simulink model "matrixMultEigenText"  (R2013b)
settings: Solver=ode3  StartTime=0.0  StopTime=10.0  FixedStep=0.001  RelTol=1e-3
InitFcn:
  | dim = 8;
  | a=randn(dim,dim);
  | matrix = ss(-a*a',randn(dim,1),randn(1,dim),0);
  | 
  | dim2 = 1;
  | dim3 = 2;
  | matA = randn(dim,dim2);
  | matC = randn(dim2,dim2);
  | matB = randn(dim2,dim3);
settings Model: Creator=rtai-ao  LastModifiedBy=rtai-ao
settings DebuggingCC: ModelReferenceIOMismatchMessage=warning
settings RTWCC: SystemTargetFile=rtai.tlc  TemplateMakefile=rtai.tmf  Description=Linux RTAI Real-Time Target  GenerateReport=on  ProcessScript=rtai_make_rtw_hook  BuildConfiguration=Faster Runs
settings STFCustomTargetCC: ModelReferenceCompliant=off  GeneratePreprocessorConditionals=Disable all  MatFileLogging=on  MATLABClassNameForMDSCustomization=Simulink.SoftwareTarget.TargetSpecificTriggerConfigurationBase  SystemTargetFile=rtai.tlc

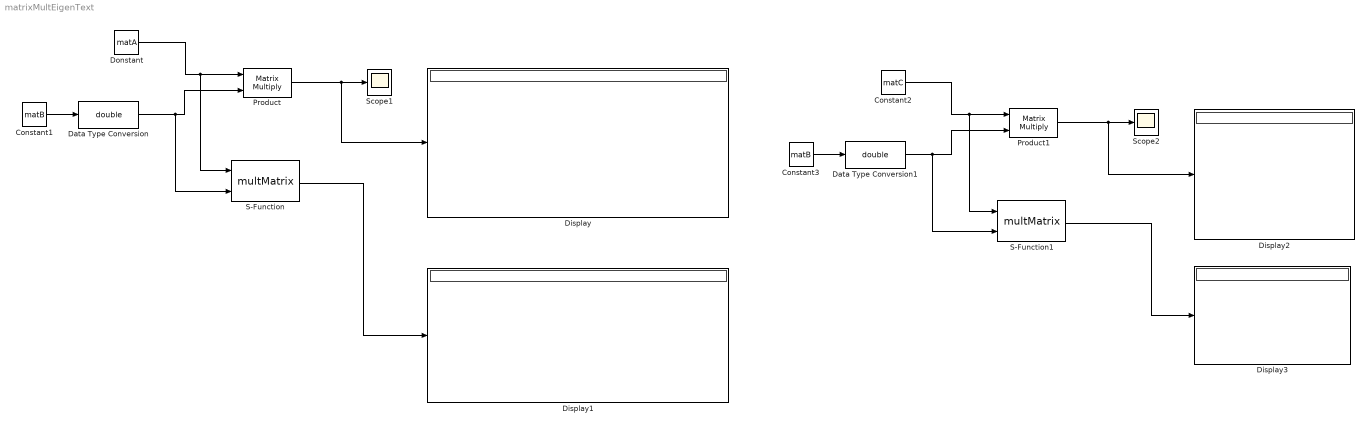
== system matrixMultEigenText ==
  Constant1 : Constant  Value=matB  VectorParams1D=off
  Constant2 : Constant  Value=matC  VectorParams1D=off
  Constant3 : Constant  Value=matB  VectorParams1D=off
  Data Type Conversion : DataTypeConversion  OutDataTypeStr=double
  Data Type Conversion1 : DataTypeConversion  OutDataTypeStr=double
  Display{,1..3} (4 alike) : Display
  Donstant : Constant  Value=matA  VectorParams1D=off
  Product : Product  Multiplication=Matrix(*)
  Product1 : Product  Multiplication=Matrix(*)
  S-Function : S-Function  RequirementInfo="{}  %GIDa_3e78427e_d73c_41cd_a138_fe399e08261f"  FunctionName=multMatrix  EnableBusSupport=off
      mask Display:
      | port_label('input',1,'A')
      | port_label('input',2,'B')
      | port_label('output',1,'Y')
      | fprintf('Y=A*B\nEigen3')
  S-Function1 : S-Function  RequirementInfo={} %GIDa_d8550f61_8f9c_4b5c_9475_fcc1fcc7cb8b  FunctionName=multMatrix  EnableBusSupport=off
      mask Display:
      | port_label('input',1,'A')
      | port_label('input',2,'B')
      | port_label('output',1,'Y')
      | fprintf('Y=A*B\nEigen3')
  Scope1 : Scope
  Scope2 : Scope
      settings: SaveName=ScopeData2
  wires:
  Product/1 -> Display/1, Scope1/1
  Constant1/1 -> Data Type Conversion/1
  Donstant/1 -> S-Function/1, Product/1
  Data Type Conversion/1 -> S-Function/2, Product/2
  Product1/1 -> Display2/1, Scope2/1
  Constant3/1 -> Data Type Conversion1/1
  S-Function1/1 -> Display3/1
  Constant2/1 -> S-Function1/1, Product1/1
  Data Type Conversion1/1 -> S-Function1/2, Product1/2
  S-Function/1 -> Display1/1
